simulink library "ThrottlePosition"  (R2024a)
settings: Solver=VariableStepAuto  StartTime=0.0  StopTime=10.0  RelTol=1e-3
undefined symbols (not defined in the file): raptor_xcp_function, StateSignal
libraries: Raptor_lib x5, Utilities x4, simulink x4
settings Model: Creator=serga  LastModifiedBy=serga

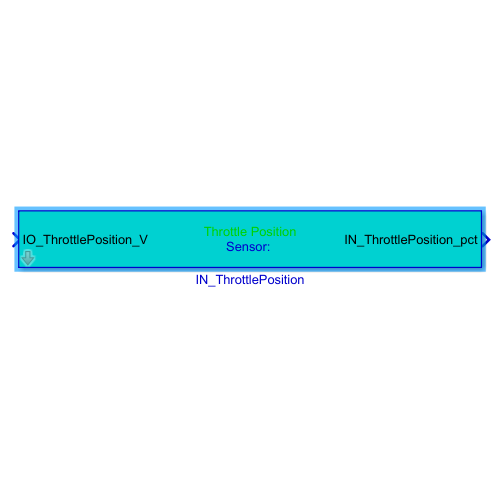
[thumbnail: Simulink's stored preview of the top-level diagram]
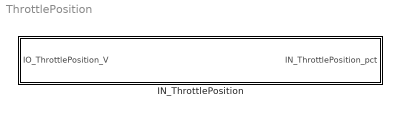
== system ThrottlePosition ==
  IN_ThrottlePosition : Subsystem  mask{pos=''}
      mask prompts: pos "Position"
      mask Display:
      | color('green')
      | disp('Throttle Position\n');
      | color('blue')
      | disp(['\nSensor: ' pos]);
      | color('black')
      | port_label('input', 1, ['IO_ThrottlePosition' pos '_V']);
      | port_label('output', 1, ['IN_ThrottlePosition' pos '_pct']);

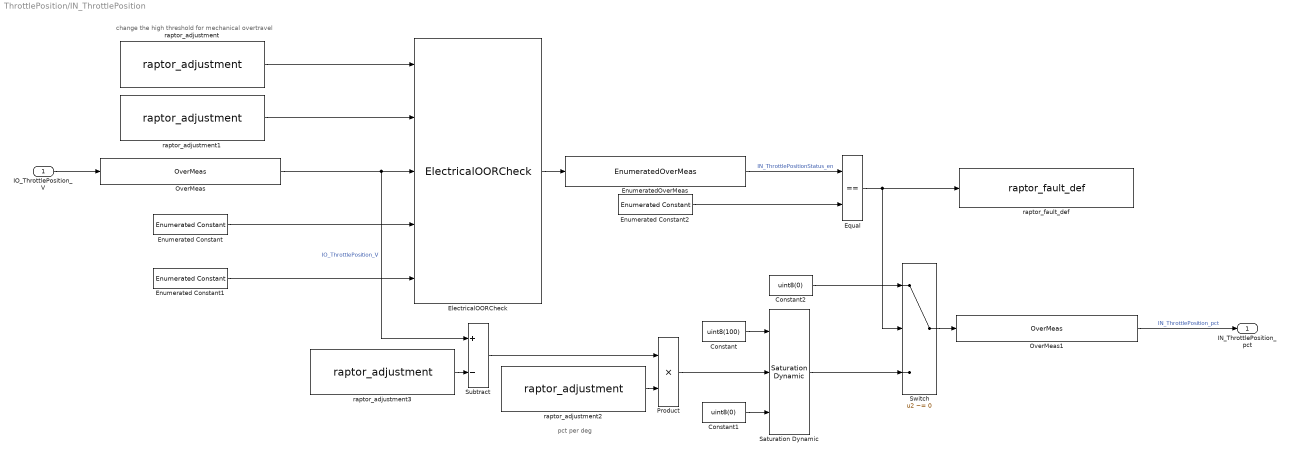
== system ThrottlePosition/IN_ThrottlePosition ==
  note: pct per deg
  note: change the high threshold for mechanical overtravel
  IO_ThrottlePosition_V : Inport
  Constant : Constant  Value=uint8(100)
  Constant1 : Constant  Value=uint8(0)
  Constant2 : Constant  Value=uint8(0)
  ElectricalOORCheck : Utilities/ElectricalOORCheck
  Enumerated Constant : simulink/Sources/Enumerated Constant  OutDataTypeStr=Enum: StateSignal  Value=StateSignal.Normal  SampleTime=inf
  Enumerated Constant1 : simulink/Sources/Enumerated Constant  OutDataTypeStr=Enum: StateSignal  Value=StateSignal.Fault  SampleTime=inf
  Enumerated Constant2 : simulink/Sources/Enumerated Constant  OutDataTypeStr=Enum: StateSignal  Value=StateSignal.Fault  SampleTime=inf
  EnumeratedOverMeas : Utilities/EnumeratedOverMeas  sigName=['IN_ThrottlePosition' pos 'Status_en']  enumName='StateSignal'
  Equal : RelationalOperator  Operator===  OutDataTypeStr=boolean  RndMeth=Simplest  InputSameDT=off
  OverMeas : Utilities/OverMeas  sigName=['IO_ThrottlePosition' pos '_V']  minimum=0  maximum=5
  OverMeas1 : Utilities/OverMeas  sigName=['IN_ThrottlePosition' pos '_pct']  minimum=0  maximum=100
  Product : Product
  Saturation Dynamic : simulink/Discontinuities/Saturation Dynamic  OutMin=[]  OutMax=[]  OutDataTypeStr=Inherit: Same as second input  OutDataType=fixdt(1, 16)  OutScaling=2^-10  DoSatur=off
  Subtract : Sum  Inputs=+-
  Switch : Switch  Criteria=u2 ~= 0  SaturateOnIntegerOverflow=off  InputSameDT=off
  raptor_adjustment : Raptor_lib/Data Storage/raptor_adjustment  paramName=['IN_ThrottlePosition' pos 'HighThresh_V']  nameSource=Parameter  initValue=4.5  dataType=single  storage=Calibration  calDispType=Number  calEnum={'False', 'True'}  calGain=1.0  calOffset=0.0  calMax=5  calMin=0  calFormat='-1'  calUnit=''  calHelp=''  calAccess=1  calFunction=raptor_xcp_function(gcb)  calDispHeaders=off  calColHeaders={'Col1' 'Col2' 'Col3'}  calRowHeaders={'Row1' 'Row2' 'Row3'}
      settings: SourceProductName=Raptor
  raptor_adjustment1 : Raptor_lib/Data Storage/raptor_adjustment  paramName=['IN_ThrottlePosition' pos 'LowThresh_V']  nameSource=Parameter  initValue=0.5  dataType=double  storage=Calibration  calDispType=Number  calEnum={'False', 'True'}  calGain=1.0  calOffset=0.0  calMax=5  calMin=0  calFormat='-1'  calUnit=''  calHelp=''  calAccess=1  calFunction=raptor_xcp_function(gcb)  calDispHeaders=off  calColHeaders={'Col1' 'Col2' 'Col3'}  calRowHeaders={'Row1' 'Row2' 'Row3'}
      settings: SourceProductName=Raptor
  raptor_adjustment2 : Raptor_lib/Data Storage/raptor_adjustment  paramName=['IN_ThrottlePosition' pos 'Scale_na']  nameSource=Parameter  initValue=5  dataType=single  storage=Calibration  calDispType=Number  calEnum={'False', 'True'}  calGain=1.0  calOffset=0.0  calMax=inf  calMin=-inf  calFormat='-1'  calUnit=''  calHelp=''  calAccess=1  calFunction=raptor_xcp_function(gcb)  calDispHeaders=off  calColHeaders={'Col1' 'Col2' 'Col3'}  calRowHeaders={'Row1' 'Row2' 'Row3'}
      settings: SourceProductName=Raptor
  raptor_adjustment3 : Raptor_lib/Data Storage/raptor_adjustment  paramName=['IN_ThrottlePosition' pos 'Zero_V']  nameSource=Parameter  initValue=2  dataType=single  storage=Calibration  calDispType=Number  calEnum={'False', 'True'}  calGain=1.0  calOffset=0.0  calMax=5  calMin=0  calFormat='-1'  calUnit=''  calHelp=''  calAccess=1  calFunction=raptor_xcp_function(gcb)  calDispHeaders=off  calColHeaders={'Col1' 'Col2' 'Col3'}  calRowHeaders={'Row1' 'Row2' 'Row3'}
      settings: SourceProductName=Raptor
  raptor_fault_def : Raptor_lib/Faults/raptor_fault_def  faultName=['IN_ThrottlePosition' pos 'Fault']  persist=off  sticky=off  emisRelated=off  singleTrip=off  clearMethod=Standard  xLimit=25  yLimit=50  calEnable=on  addDisable=off  calAccess=1  calFunction='System | FaultManager'
      settings: SourceProductName=Raptor
  IN_ThrottlePosition_pct : Outport
  wires:
  Switch/1 -> OverMeas1/1
  OverMeas1/1 -> IN_ThrottlePosition_pct/1  "IN_ThrottlePosition_pct"
  Constant2/1 -> Switch/1
  Constant1/1 -> Saturation Dynamic/3
  Constant/1 -> Saturation Dynamic/1
  Saturation Dynamic/1 -> Switch/3
  Product/1 -> Saturation Dynamic/2
  Subtract/1 -> Product/1
  raptor_adjustment3/1 -> Subtract/2
  raptor_adjustment2/1 -> Product/2
  EnumeratedOverMeas/1 -> Equal/1  "IN_ThrottlePositionStatus_en"
  Equal/1 -> raptor_fault_def/1, Switch/2
  Enumerated Constant2/1 -> Equal/2
  ElectricalOORCheck/1 -> EnumeratedOverMeas/1
  Enumerated Constant1/1 -> ElectricalOORCheck/5
  Enumerated Constant/1 -> ElectricalOORCheck/4
  raptor_adjustment1/1 -> ElectricalOORCheck/2
  raptor_adjustment/1 -> ElectricalOORCheck/1
  OverMeas/1 -> ElectricalOORCheck/3, Subtract/1  "IO_ThrottlePosition_V"
  IO_ThrottlePosition_V/1 -> OverMeas/1
